simulink model "Stabilization_simulink_linear"  (R2025b)
settings: Solver=ode4  StartTime=0.0  StopTime=1  FixedStep=1/200  RelTol=1e-3
undefined symbols (not defined in the file or in its folder): input_deg, Ki, Km, Kp, Pm
settings Model: Creator=chaeeun  LastModifiedBy=ADMIN

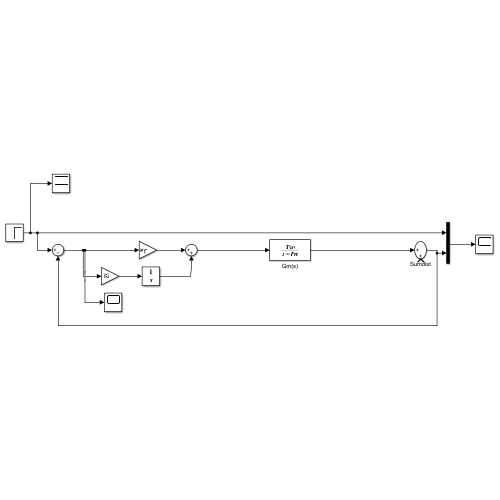
[thumbnail: Simulink's stored preview of the top-level diagram]
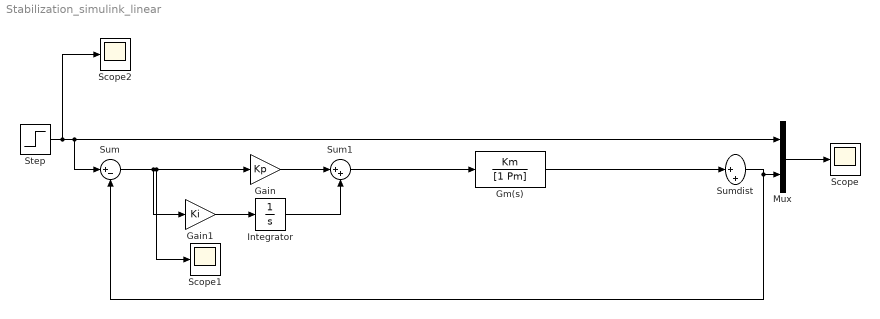
== system Stabilization_simulink_linear ==
  Gain : Gain  Gain=Kp
  Gain1 : Gain  Gain=Ki
  Gm(s) : TransferFcn  Numerator=Km  Denominator=[1 Pm]
  Integrator : Integrator
  Mux : Mux  Inputs=2
  Scope : Scope
      settings: ActiveDisplayYMinimum=0.87681641914079655  ActiveDisplayYMaximum=7.9623882696898249
  Scope1 : Scope
      settings: ActiveDisplayYMinimum=-1  ActiveDisplayYMaximum=1
  Scope2 : Scope
      settings: ActiveDisplayYMinimum=-1  ActiveDisplayYMaximum=1  DataLoggingVariableName=ScopeData2
  Step : Step  Time=0  After=input_deg  SampleTime=0  VectorParams1D=off
  Sum : Sum  Inputs=|+-
  Sum1 : Sum  Inputs=|++
  Sumdist : Sum  Inputs=|++
  wires:
  Sumdist/1 -> Sum/2, Mux/2
  Mux/1 -> Scope/1
  Step/1 -> Scope2/1, Mux/1, Sum/1
  Gain/1 -> Sum1/1
  Sum/1 -> Gain/1, Scope1/1, Gain1/1
  Gain1/1 -> Integrator/1
  Integrator/1 -> Sum1/2
  Sum1/1 -> Gm(s)/1
  Gm(s)/1 -> Sumdist/1
